simulink model "TST_DevLib_ActrPrt"  (R2016b)
settings: Solver=FixedStepDiscrete  StartTime=0.0  StopTime=simTime  FixedStep=sampleTime  RelTol=1e-3
values from neighbouring files (symbols this model uses):
  testCase = 1    [initTST_DevLib_ActrPrt_001.m]    (also in initTST_DevLib_ActrPrt_002.m = 2; initTST_DevLib_ActrPrt_003.m = 3)
libraries: simulink x7, UnitTest_Lib x3
settings Model: Creator=zhengjinyan  LastModifiedBy=zhengjinyan
settings DebuggingCC: SignalRangeChecking=error

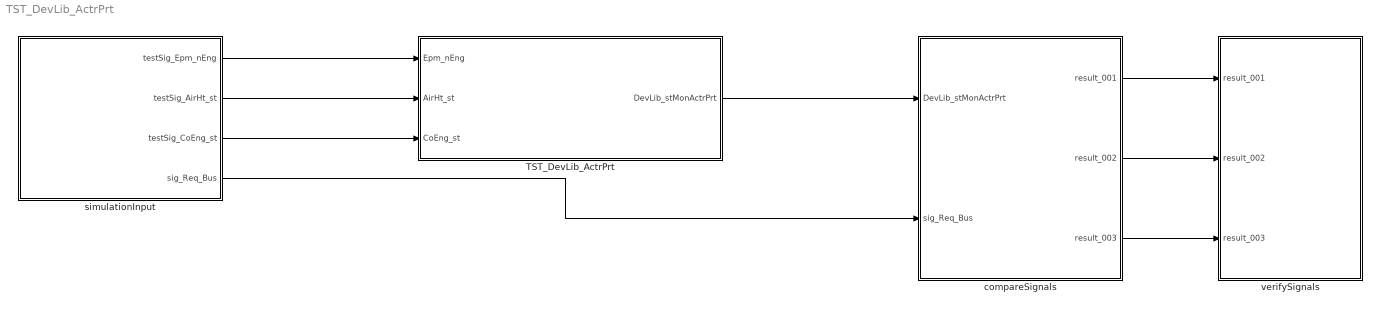
== system TST_DevLib_ActrPrt ==
  TST_DevLib_ActrPrt : Subsystem
  compareSignals : Subsystem
  simulationInput : Subsystem
  verifySignals : Subsystem
  wires:
  simulationInput/1(testSig_Epm_nEng) -> TST_DevLib_ActrPrt/1(Epm_nEng)
  simulationInput/2(testSig_AirHt_st) -> TST_DevLib_ActrPrt/2(AirHt_st)
  simulationInput/3(testSig_CoEng_st) -> TST_DevLib_ActrPrt/3(CoEng_st)
  TST_DevLib_ActrPrt/1(DevLib_stMonActrPrt) -> compareSignals/1(DevLib_stMonActrPrt)
  simulationInput/4(sig_Req_Bus) -> compareSignals/2(sig_Req_Bus)
  compareSignals/1(result_001) -> verifySignals/1(result_001)
  compareSignals/2(result_002) -> verifySignals/2(result_002)
  compareSignals/3(result_003) -> verifySignals/3(result_003)

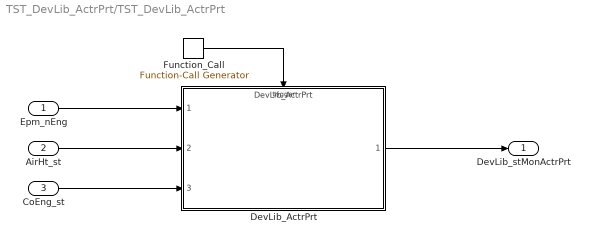
== system TST_DevLib_ActrPrt/TST_DevLib_ActrPrt ==
  Epm_nEng : Inport
  AirHt_st : Inport  Port=2
  CoEng_st : Inport  Port=3
  DevLib_ActrPrt : ModelReference  ModelNameDialog=DevLib_ActrPrt  SimulationMode=Normal  ModelReferenceVersion=1.7  TriggerPortName=function  TriggerPortTriggerType=function-call  TriggerPortStatesWhenEnabling=held
  Function_Call : simulink/Ports & Subsystems/Function-Call Generator  sample_time=sampleTime  numberOfIterations=1
  DevLib_stMonActrPrt : Outport
  wires:
  Function_Call/1 -> DevLib_ActrPrt/Trigger
  Epm_nEng/1 -> DevLib_ActrPrt/1
  AirHt_st/1 -> DevLib_ActrPrt/2
  CoEng_st/1 -> DevLib_ActrPrt/3
  DevLib_ActrPrt/1 -> DevLib_stMonActrPrt/1

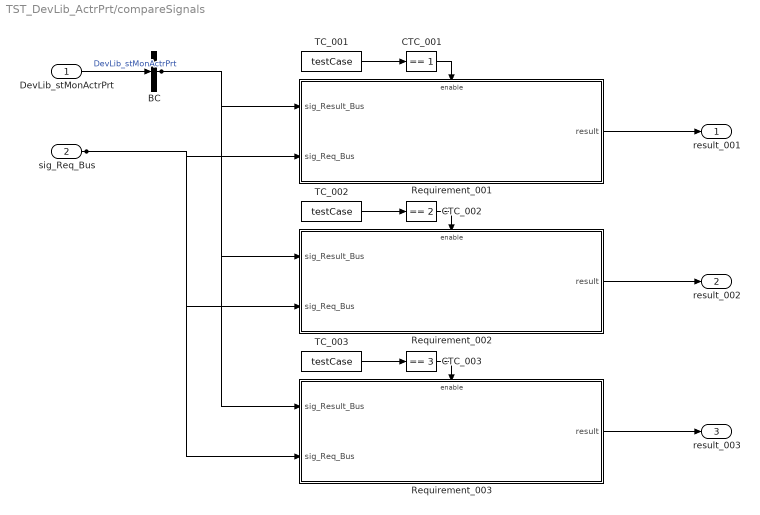
== system TST_DevLib_ActrPrt/compareSignals ==
  DevLib_stMonActrPrt : Inport
  sig_Req_Bus : Inport  Port=2
  BC : BusCreator  Inputs=1
  CTC_001 : simulink/Logic and Bit Operations/Compare To Constant  relop===  const=1  OutDataTypeStr=boolean
  CTC_002 : simulink/Logic and Bit Operations/Compare To Constant  relop===  const=2  OutDataTypeStr=boolean
  CTC_003 : simulink/Logic and Bit Operations/Compare To Constant  relop===  const=3  OutDataTypeStr=boolean
  Requirement_001 : Subsystem
  Requirement_002 : Subsystem
  Requirement_003 : Subsystem
  TC_001 : Constant  Value=testCase
  TC_002 : Constant  Value=testCase
  TC_003 : Constant  Value=testCase
  result_001 : Outport
  result_002 : Outport  Port=2
  result_003 : Outport  Port=3
  wires:
  DevLib_stMonActrPrt/1 -> BC/1  "DevLib_stMonActrPrt"
  TC_001/1 -> CTC_001/1
  CTC_001/1 -> Requirement_001/Enable
  sig_Req_Bus/1 -> Requirement_001/2(sig_Req_Bus), Requirement_002/2(sig_Req_Bus), Requirement_003/2(sig_Req_Bus)
  BC/1 -> Requirement_001/1(sig_Result_Bus), Requirement_002/1(sig_Result_Bus), Requirement_003/1(sig_Result_Bus)
  Requirement_001/1(result) -> result_001/1
  TC_002/1 -> CTC_002/1
  CTC_002/1 -> Requirement_002/Enable
  Requirement_002/1(result) -> result_002/1
  TC_003/1 -> CTC_003/1
  CTC_003/1 -> Requirement_003/Enable
  Requirement_003/1(result) -> result_003/1

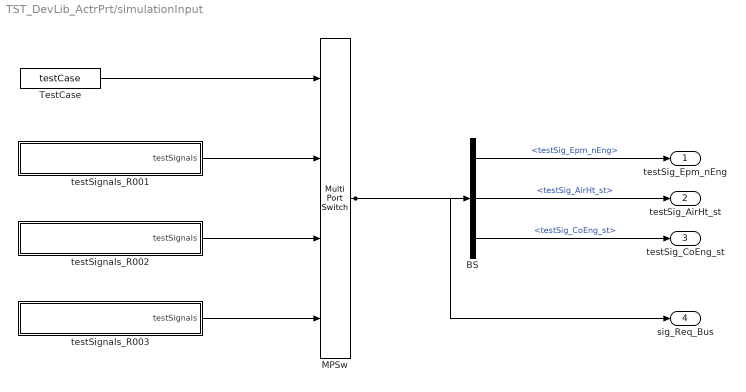
== system TST_DevLib_ActrPrt/simulationInput ==
  BS : BusSelector  OutputSignals=testSig_Epm_nEng,testSig_AirHt_st,testSig_CoEng_st
  MPSw : MultiPortSwitch  SaturateOnIntegerOverflow=on  InputSameDT=on
  TestCase : Constant  Value=testCase
  testSignals_R001 : Subsystem
  testSignals_R002 : Subsystem
  testSignals_R003 : Subsystem
  testSig_Epm_nEng : Outport
  testSig_AirHt_st : Outport  Port=2
  testSig_CoEng_st : Outport  Port=3
  sig_Req_Bus : Outport  Port=4
  wires:
  BS/1 -> testSig_Epm_nEng/1  "<testSig_Epm_nEng>"
  BS/2 -> testSig_AirHt_st/1  "<testSig_AirHt_st>"
  BS/3 -> testSig_CoEng_st/1  "<testSig_CoEng_st>"
  MPSw/1 -> BS/1, sig_Req_Bus/1
  TestCase/1 -> MPSw/1
  testSignals_R001/1(testSignals) -> MPSw/2
  testSignals_R002/1(testSignals) -> MPSw/3
  testSignals_R003/1(testSignals) -> MPSw/4

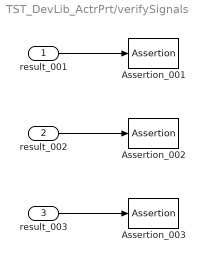
== system TST_DevLib_ActrPrt/verifySignals ==
  result_001 : Inport
  result_002 : Inport  Port=2
  result_003 : Inport  Port=3
  Assertion_001 : Assertion  Enabled=off
  Assertion_002 : Assertion  Enabled=off
  Assertion_003 : Assertion  Enabled=off
  wires:
  result_001/1 -> Assertion_001/1
  result_002/1 -> Assertion_002/1
  result_003/1 -> Assertion_003/1

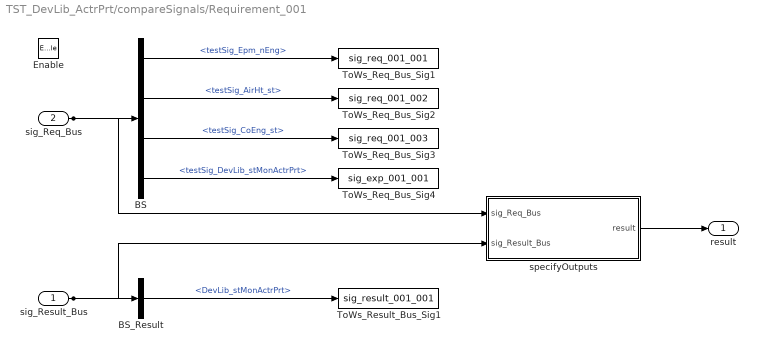
== system TST_DevLib_ActrPrt/compareSignals/Requirement_001 ==
  sig_Result_Bus : Inport
  sig_Req_Bus : Inport  Port=2
  Enable : EnablePort
  BS : BusSelector  OutputSignals=testSig_Epm_nEng,testSig_AirHt_st,testSig_CoEng_st,testSig_DevLib_stMonActrPrt
  BS_Result : BusSelector  OutputSignals=DevLib_stMonActrPrt
  ToWs_Req_Bus_Sig1 : ToWorkspace  VariableName=sig_req_001_001  SaveFormat=Structure With Time
  ToWs_Req_Bus_Sig2 : ToWorkspace  VariableName=sig_req_001_002  SaveFormat=Structure With Time
  ToWs_Req_Bus_Sig3 : ToWorkspace  VariableName=sig_req_001_003  SaveFormat=Structure With Time
  ToWs_Req_Bus_Sig4 : ToWorkspace  VariableName=sig_exp_001_001  SaveFormat=Structure With Time
  ToWs_Result_Bus_Sig1 : ToWorkspace  VariableName=sig_result_001_001  SaveFormat=Structure With Time
  specifyOutputs : Subsystem
  result : Outport
  wires:
  sig_Req_Bus/1 -> BS/1, specifyOutputs/1(sig_Req_Bus)
  BS/1 -> ToWs_Req_Bus_Sig1/1  "<testSig_Epm_nEng>"
  BS/2 -> ToWs_Req_Bus_Sig2/1  "<testSig_AirHt_st>"
  BS/3 -> ToWs_Req_Bus_Sig3/1  "<testSig_CoEng_st>"
  BS/4 -> ToWs_Req_Bus_Sig4/1  "<testSig_DevLib_stMonActrPrt>"
  sig_Result_Bus/1 -> BS_Result/1, specifyOutputs/2(sig_Result_Bus)
  BS_Result/1 -> ToWs_Result_Bus_Sig1/1  "<DevLib_stMonActrPrt>"
  specifyOutputs/1(result) -> result/1

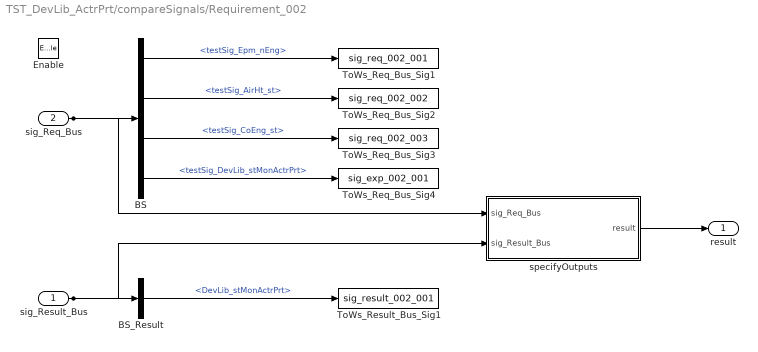
== system TST_DevLib_ActrPrt/compareSignals/Requirement_002 ==
  sig_Result_Bus : Inport
  sig_Req_Bus : Inport  Port=2
  Enable : EnablePort
  BS : BusSelector  OutputSignals=testSig_Epm_nEng,testSig_AirHt_st,testSig_CoEng_st,testSig_DevLib_stMonActrPrt
  BS_Result : BusSelector  OutputSignals=DevLib_stMonActrPrt
  ToWs_Req_Bus_Sig1 : ToWorkspace  VariableName=sig_req_002_001  SaveFormat=Structure With Time
  ToWs_Req_Bus_Sig2 : ToWorkspace  VariableName=sig_req_002_002  SaveFormat=Structure With Time
  ToWs_Req_Bus_Sig3 : ToWorkspace  VariableName=sig_req_002_003  SaveFormat=Structure With Time
  ToWs_Req_Bus_Sig4 : ToWorkspace  VariableName=sig_exp_002_001  SaveFormat=Structure With Time
  ToWs_Result_Bus_Sig1 : ToWorkspace  VariableName=sig_result_002_001  SaveFormat=Structure With Time
  specifyOutputs : Subsystem
  result : Outport
  wires:
  sig_Req_Bus/1 -> BS/1, specifyOutputs/1(sig_Req_Bus)
  BS/1 -> ToWs_Req_Bus_Sig1/1  "<testSig_Epm_nEng>"
  BS/2 -> ToWs_Req_Bus_Sig2/1  "<testSig_AirHt_st>"
  BS/3 -> ToWs_Req_Bus_Sig3/1  "<testSig_CoEng_st>"
  BS/4 -> ToWs_Req_Bus_Sig4/1  "<testSig_DevLib_stMonActrPrt>"
  sig_Result_Bus/1 -> BS_Result/1, specifyOutputs/2(sig_Result_Bus)
  BS_Result/1 -> ToWs_Result_Bus_Sig1/1  "<DevLib_stMonActrPrt>"
  specifyOutputs/1(result) -> result/1

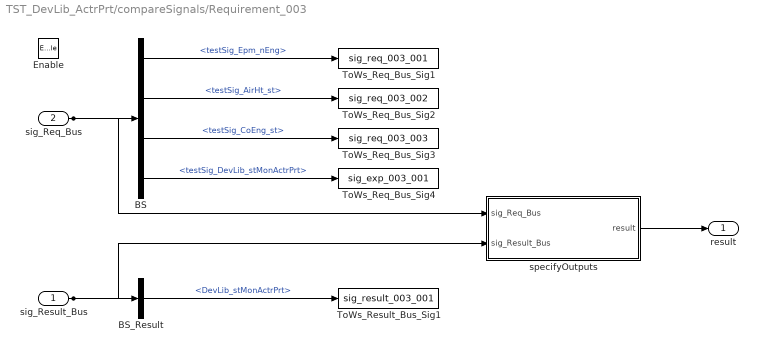
== system TST_DevLib_ActrPrt/compareSignals/Requirement_003 ==
  sig_Result_Bus : Inport
  sig_Req_Bus : Inport  Port=2
  Enable : EnablePort
  BS : BusSelector  OutputSignals=testSig_Epm_nEng,testSig_AirHt_st,testSig_CoEng_st,testSig_DevLib_stMonActrPrt
  BS_Result : BusSelector  OutputSignals=DevLib_stMonActrPrt
  ToWs_Req_Bus_Sig1 : ToWorkspace  VariableName=sig_req_003_001  SaveFormat=Structure With Time
  ToWs_Req_Bus_Sig2 : ToWorkspace  VariableName=sig_req_003_002  SaveFormat=Structure With Time
  ToWs_Req_Bus_Sig3 : ToWorkspace  VariableName=sig_req_003_003  SaveFormat=Structure With Time
  ToWs_Req_Bus_Sig4 : ToWorkspace  VariableName=sig_exp_003_001  SaveFormat=Structure With Time
  ToWs_Result_Bus_Sig1 : ToWorkspace  VariableName=sig_result_003_001  SaveFormat=Structure With Time
  specifyOutputs : Subsystem
  result : Outport
  wires:
  sig_Req_Bus/1 -> BS/1, specifyOutputs/1(sig_Req_Bus)
  BS/1 -> ToWs_Req_Bus_Sig1/1  "<testSig_Epm_nEng>"
  BS/2 -> ToWs_Req_Bus_Sig2/1  "<testSig_AirHt_st>"
  BS/3 -> ToWs_Req_Bus_Sig3/1  "<testSig_CoEng_st>"
  BS/4 -> ToWs_Req_Bus_Sig4/1  "<testSig_DevLib_stMonActrPrt>"
  sig_Result_Bus/1 -> BS_Result/1, specifyOutputs/2(sig_Result_Bus)
  BS_Result/1 -> ToWs_Result_Bus_Sig1/1  "<DevLib_stMonActrPrt>"
  specifyOutputs/1(result) -> result/1

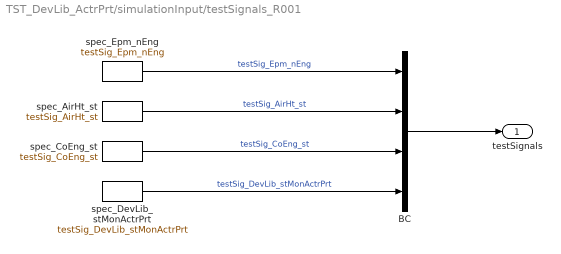
== system TST_DevLib_ActrPrt/simulationInput/testSignals_R001 ==
  BC : BusCreator  Inputs=4
  spec_AirHt_st : FromWorkspace  VariableName=testSig_AirHt_st  Interpolate=off  OutputAfterFinalValue=Holding final value
  spec_CoEng_st : FromWorkspace  VariableName=testSig_CoEng_st  Interpolate=off  OutputAfterFinalValue=Holding final value
  spec_DevLib_stMonActrPrt : FromWorkspace  VariableName=testSig_DevLib_stMonActrPrt  Interpolate=off  OutputAfterFinalValue=Holding final value
  spec_Epm_nEng : FromWorkspace  VariableName=testSig_Epm_nEng  Interpolate=off  OutputAfterFinalValue=Holding final value
  testSignals : Outport
  wires:
  BC/1 -> testSignals/1
  spec_Epm_nEng/1 -> BC/1  "testSig_Epm_nEng"
  spec_AirHt_st/1 -> BC/2  "testSig_AirHt_st"
  spec_CoEng_st/1 -> BC/3  "testSig_CoEng_st"
  spec_DevLib_stMonActrPrt/1 -> BC/4  "testSig_DevLib_stMonActrPrt"

== system TST_DevLib_ActrPrt/simulationInput/testSignals_R002 ==
  BC : BusCreator  Inputs=4
  spec_AirHt_st : FromWorkspace  VariableName=testSig_AirHt_st  Interpolate=off  OutputAfterFinalValue=Holding final value
  spec_CoEng_st : FromWorkspace  VariableName=testSig_CoEng_st  Interpolate=off  OutputAfterFinalValue=Holding final value
  spec_DevLib_stMonActrPrt : FromWorkspace  VariableName=testSig_DevLib_stMonActrPrt  Interpolate=off  OutputAfterFinalValue=Holding final value
  spec_Epm_nEng : FromWorkspace  VariableName=testSig_Epm_nEng  Interpolate=off  OutputAfterFinalValue=Holding final value
  testSignals : Outport
  wires:
  BC/1 -> testSignals/1
  spec_Epm_nEng/1 -> BC/1  "testSig_Epm_nEng"
  spec_AirHt_st/1 -> BC/2  "testSig_AirHt_st"
  spec_CoEng_st/1 -> BC/3  "testSig_CoEng_st"
  spec_DevLib_stMonActrPrt/1 -> BC/4  "testSig_DevLib_stMonActrPrt"

== system TST_DevLib_ActrPrt/simulationInput/testSignals_R003 ==
  BC : BusCreator  Inputs=4
  spec_AirHt_st : FromWorkspace  VariableName=testSig_AirHt_st  Interpolate=off  OutputAfterFinalValue=Holding final value
  spec_CoEng_st : FromWorkspace  VariableName=testSig_CoEng_st  Interpolate=off  OutputAfterFinalValue=Holding final value
  spec_DevLib_stMonActrPrt : FromWorkspace  VariableName=testSig_DevLib_stMonActrPrt  Interpolate=off  OutputAfterFinalValue=Holding final value
  spec_Epm_nEng : FromWorkspace  VariableName=testSig_Epm_nEng  Interpolate=off  OutputAfterFinalValue=Holding final value
  testSignals : Outport
  wires:
  BC/1 -> testSignals/1
  spec_Epm_nEng/1 -> BC/1  "testSig_Epm_nEng"
  spec_AirHt_st/1 -> BC/2  "testSig_AirHt_st"
  spec_CoEng_st/1 -> BC/3  "testSig_CoEng_st"
  spec_DevLib_stMonActrPrt/1 -> BC/4  "testSig_DevLib_stMonActrPrt"

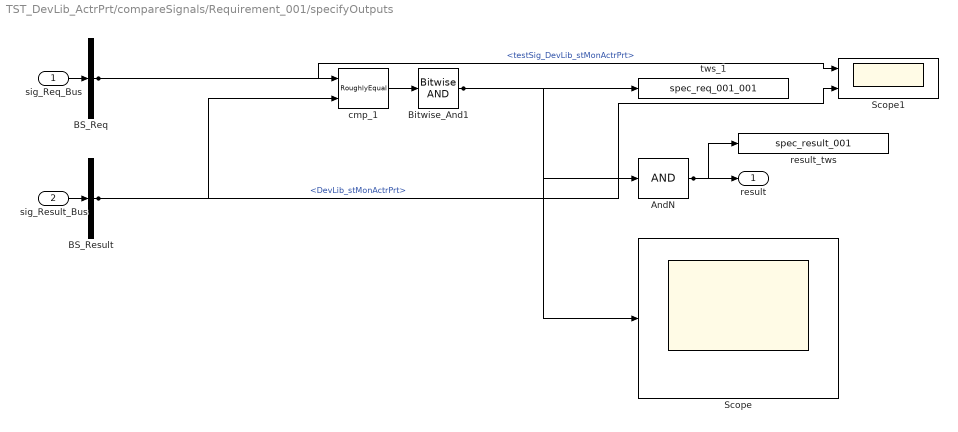
== system TST_DevLib_ActrPrt/compareSignals/Requirement_001/specifyOutputs ==
  sig_Req_Bus : Inport
  sig_Result_Bus : Inport  Port=2
  AndN : Logic  Inputs=1
  BS_Req : BusSelector  OutputSignals=testSig_DevLib_stMonActrPrt
  BS_Result : BusSelector  OutputSignals=DevLib_stMonActrPrt
  Bitwise_And1 : simulink/Logic and Bit Operations/Bitwise Operator  logicop=AND  UseBitMask=off  BitMask=bin2dec('11011001')  BitMaskRealWorld=Stored Integer
  Scope : Scope
  Scope1 : Scope  NumInputPorts=2
  cmp_1 : UnitTest_Lib/RoughlyEqual  slope=0.1
  result_tws : ToWorkspace  VariableName=spec_result_001
  tws_1 : ToWorkspace  VariableName=spec_req_001_001
  result : Outport
  wires:
  sig_Req_Bus/1 -> BS_Req/1
  sig_Result_Bus/1 -> BS_Result/1
  AndN/1 -> result/1, result_tws/1
  BS_Req/1 -> cmp_1/1, Scope1/1  "<testSig_DevLib_stMonActrPrt>"
  BS_Result/1 -> cmp_1/2, Scope1/2  "<DevLib_stMonActrPrt>"
  cmp_1/1 -> Bitwise_And1/1
  Bitwise_And1/1 -> tws_1/1, AndN/1, Scope/1

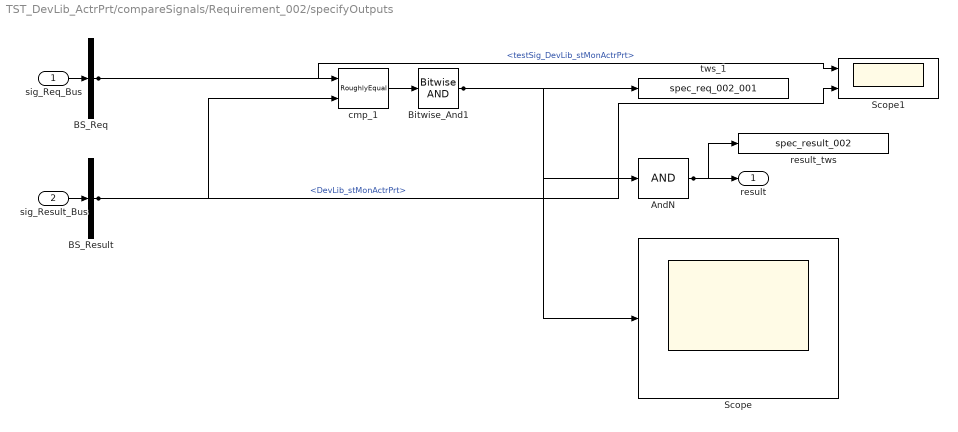
== system TST_DevLib_ActrPrt/compareSignals/Requirement_002/specifyOutputs ==
  sig_Req_Bus : Inport
  sig_Result_Bus : Inport  Port=2
  AndN : Logic  Inputs=1
  BS_Req : BusSelector  OutputSignals=testSig_DevLib_stMonActrPrt
  BS_Result : BusSelector  OutputSignals=DevLib_stMonActrPrt
  Bitwise_And1 : simulink/Logic and Bit Operations/Bitwise Operator  logicop=AND  UseBitMask=off  BitMask=bin2dec('11011001')  BitMaskRealWorld=Stored Integer
  Scope : Scope
  Scope1 : Scope  NumInputPorts=2
  cmp_1 : UnitTest_Lib/RoughlyEqual  slope=0.1
  result_tws : ToWorkspace  VariableName=spec_result_002
  tws_1 : ToWorkspace  VariableName=spec_req_002_001
  result : Outport
  wires:
  sig_Req_Bus/1 -> BS_Req/1
  sig_Result_Bus/1 -> BS_Result/1
  AndN/1 -> result/1, result_tws/1
  BS_Req/1 -> cmp_1/1, Scope1/1  "<testSig_DevLib_stMonActrPrt>"
  BS_Result/1 -> cmp_1/2, Scope1/2  "<DevLib_stMonActrPrt>"
  cmp_1/1 -> Bitwise_And1/1
  Bitwise_And1/1 -> tws_1/1, AndN/1, Scope/1

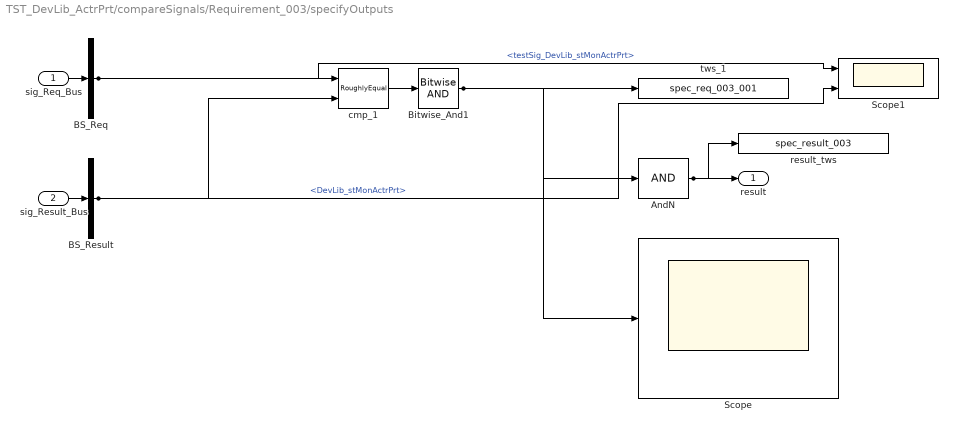
== system TST_DevLib_ActrPrt/compareSignals/Requirement_003/specifyOutputs ==
  sig_Req_Bus : Inport
  sig_Result_Bus : Inport  Port=2
  AndN : Logic  Inputs=1
  BS_Req : BusSelector  OutputSignals=testSig_DevLib_stMonActrPrt
  BS_Result : BusSelector  OutputSignals=DevLib_stMonActrPrt
  Bitwise_And1 : simulink/Logic and Bit Operations/Bitwise Operator  logicop=AND  UseBitMask=off  BitMask=bin2dec('11011001')  BitMaskRealWorld=Stored Integer
  Scope : Scope
  Scope1 : Scope  NumInputPorts=2
  cmp_1 : UnitTest_Lib/RoughlyEqual  slope=0.1
  result_tws : ToWorkspace  VariableName=spec_result_003
  tws_1 : ToWorkspace  VariableName=spec_req_003_001
  result : Outport
  wires:
  sig_Req_Bus/1 -> BS_Req/1
  sig_Result_Bus/1 -> BS_Result/1
  AndN/1 -> result/1, result_tws/1
  BS_Req/1 -> cmp_1/1, Scope1/1  "<testSig_DevLib_stMonActrPrt>"
  BS_Result/1 -> cmp_1/2, Scope1/2  "<DevLib_stMonActrPrt>"
  cmp_1/1 -> Bitwise_And1/1
  Bitwise_And1/1 -> tws_1/1, AndN/1, Scope/1
